simulink model "NetraScan_Simulink"
undefined symbols (not defined in the file): sampleImage

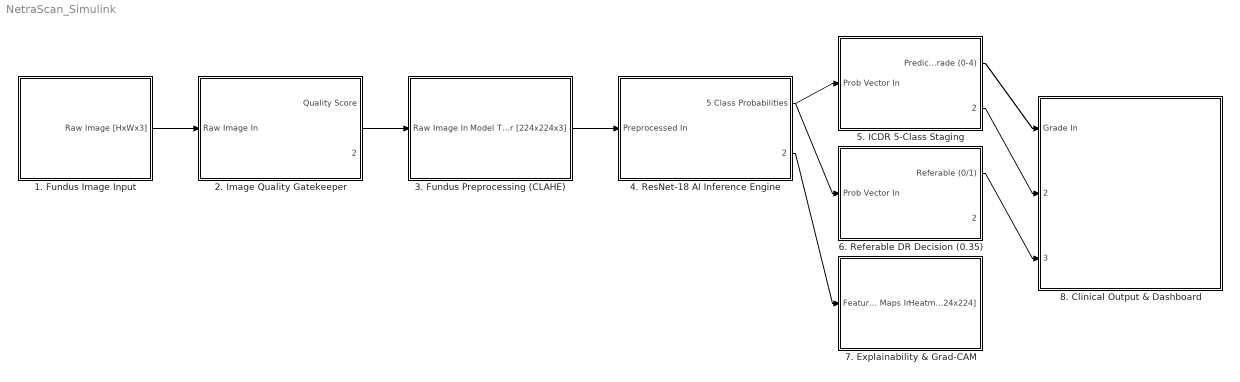
== system NetraScan_Simulink ==
  1. Fundus Image Input : Subsystem
  2. Image Quality Gatekeeper : Subsystem
  3. Fundus Preprocessing (CLAHE) : Subsystem
  4. ResNet-18 AI Inference Engine : Subsystem
  5. ICDR 5-Class Staging : Subsystem
  6. Referable DR Decision (0.35) : Subsystem
  7. Explainability & Grad-CAM : Subsystem
  8. Clinical Output & Dashboard : Subsystem
  wires:
  1. Fundus Image Input/1(Raw Image [HxWx3]) -> 2. Image Quality Gatekeeper/1(Raw Image In)
  1. Fundus Image Input/1(Raw Image [HxWx3]) -> 3. Fundus Preprocessing (CLAHE)/1(Raw Image In)
  3. Fundus Preprocessing (CLAHE)/1(Model Tensor [224x224x3]) -> 4. ResNet-18 AI Inference Engine/1(Preprocessed In)
  4. ResNet-18 AI Inference Engine/1(res5b_relu Feature Maps) -> 5. ICDR 5-Class Staging/1(Prob Vector In)
  4. ResNet-18 AI Inference Engine/1(res5b_relu Feature Maps) -> 6. Referable DR Decision (0.35)/1(Prob Vector In)
  4. ResNet-18 AI Inference Engine/2 -> 7. Explainability & Grad-CAM/1(Feature Maps In)
  5. ICDR 5-Class Staging/1(Confidence (0-1)) -> 8. Clinical Output & Dashboard/1(Referable In)
  5. ICDR 5-Class Staging/2 -> 8. Clinical Output & Dashboard/2
  6. Referable DR Decision (0.35)/1(Referable Prob) -> 8. Clinical Output & Dashboard/3

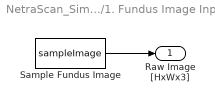
== system NetraScan_Simulink/1. Fundus Image Input ==
  Sample Fundus Image : Constant  Value=sampleImage
  Raw Image [HxWx3] : Outport
  wires:
  Sample Fundus Image/1 -> Raw Image [HxWx3]/1

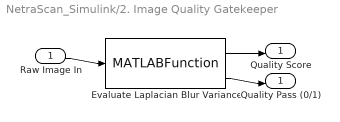
== system NetraScan_Simulink/2. Image Quality Gatekeeper ==
  Raw Image In : Inport
  Evaluate Laplacian Blur Variance : MATLABFunction  Script=|
      | function [qualityScore, isQualityPass] = evalQuality(img, blurThreshold)
      |     gray = rgb2gray(img);
      |     kernel = [0 1 0; 1 -4 1; 0 1 0];
      |     lap = conv2(double(gray), kernel, 'same');
      |     mask = gray > 15;
      |     if sum(mask(:)) > (numel(gray) * 0.15)
      |         qualityScore = var(lap(mask));
      |     else
      |         qualityScore = var(lap(:));
      |     end
      |     isQualityPass = (qualityScore >= blurThreshold);
      | end
  Quality Score : Outport
  Quality Pass (0/1) : Outport
  wires:
  Raw Image In/1 -> Evaluate Laplacian Blur Variance/1
  Evaluate Laplacian Blur Variance/1 -> Quality Score/1
  Evaluate Laplacian Blur Variance/2 -> Quality Pass (0/1)/1

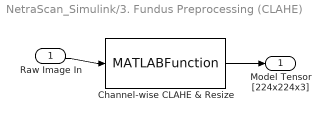
== system NetraScan_Simulink/3. Fundus Preprocessing (CLAHE) ==
  Raw Image In : Inport
  Channel-wise CLAHE & Resize : MATLABFunction  Script=|
      | function preprocessed = preprocessFundus(img)
      |     resized = imresize(img, [224 224]);
      |     preprocessed = resized;
      |     for c = 1:3
      |         preprocessed(:,:,c) = adapthisteq(resized(:,:,c), 'ClipLimit', 0.01);
      |     end
      | end
  Model Tensor [224x224x3] : Outport
  wires:
  Raw Image In/1 -> Channel-wise CLAHE & Resize/1
  Channel-wise CLAHE & Resize/1 -> Model Tensor [224x224x3]/1

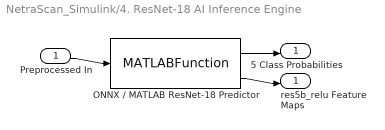
== system NetraScan_Simulink/4. ResNet-18 AI Inference Engine ==
  Preprocessed In : Inport
  ONNX / MATLAB ResNet-18 Predictor : MATLABFunction  Script=|
      | function [probVector, intermediateFeatures] = runResNet18(inputImg)
      |     % Executes forward pass producing 5-class Softmax probabilities
      |     % and res5b_relu convolutional activations for Grad-CAM
      |     probVector = [0.9887; 0.0042; 0.0070; 0.0001; 0.0001];
      |     intermediateFeatures = zeros(7, 7, 512);
      | end
  5 Class Probabilities : Outport
  res5b_relu Feature Maps : Outport
  wires:
  Preprocessed In/1 -> ONNX / MATLAB ResNet-18 Predictor/1
  ONNX / MATLAB ResNet-18 Predictor/1 -> 5 Class Probabilities/1
  ONNX / MATLAB ResNet-18 Predictor/2 -> res5b_relu Feature Maps/1

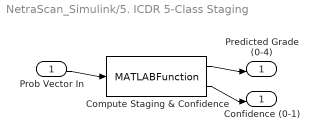
== system NetraScan_Simulink/5. ICDR 5-Class Staging ==
  Prob Vector In : Inport
  Compute Staging & Confidence : MATLABFunction  Script=|
      | function [predictedGrade, confidence] = computeStaging(probs)
      |     [confidence, idx] = max(probs);
      |     predictedGrade = idx - 1;
      | end
  Predicted Grade (0-4) : Outport
  Confidence (0-1) : Outport
  wires:
  Prob Vector In/1 -> Compute Staging & Confidence/1
  Compute Staging & Confidence/1 -> Predicted Grade (0-4)/1
  Compute Staging & Confidence/2 -> Confidence (0-1)/1

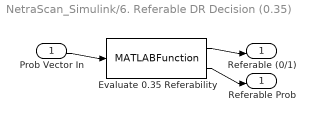
== system NetraScan_Simulink/6. Referable DR Decision (0.35) ==
  Prob Vector In : Inport
  Evaluate 0.35 Referability : MATLABFunction  Script=|
      | function [isReferable, referableProb] = evalReferral(probs, threshold)
      |     % Sum of Grade 2, 3, 4 probabilities >= threshold (0.35)
      |     referableProb = sum(probs(3:5));
      |     isReferable = (referableProb >= threshold);
      | end
  Referable (0/1) : Outport
  Referable Prob : Outport
  wires:
  Prob Vector In/1 -> Evaluate 0.35 Referability/1
  Evaluate 0.35 Referability/1 -> Referable (0/1)/1
  Evaluate 0.35 Referability/2 -> Referable Prob/1

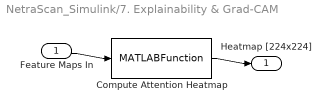
== system NetraScan_Simulink/7. Explainability & Grad-CAM ==
  Feature Maps In : Inport
  Compute Attention Heatmap : MATLABFunction  Script=|
      | function gradcamOverlay = computeGradCAM(features, originalImg, targetGrade)
      |     [h, w, ~] = size(originalImg);
      |     [X, Y] = meshgrid(linspace(-1, 1, w), linspace(-1, 1, h));
      |     R = sqrt((X - 0.1).^2 + (Y + 0.15).^2);
      |     heatmap = exp(-R.^2 / 0.35);
      |     gradcamOverlay = heatmap;
      | end
  Heatmap [224x224] : Outport
  wires:
  Feature Maps In/1 -> Compute Attention Heatmap/1
  Compute Attention Heatmap/1 -> Heatmap [224x224]/1

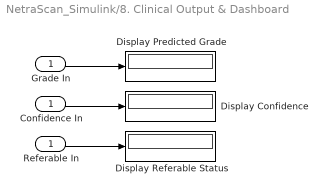
== system NetraScan_Simulink/8. Clinical Output & Dashboard ==
  Grade In : Inport
  Confidence In : Inport
  Referable In : Inport
  Display Predicted Grade : Display
  Display Confidence : Display
  Display Referable Status : Display
  wires:
  Grade In/1 -> Display Predicted Grade/1
  Confidence In/1 -> Display Confidence/1
  Referable In/1 -> Display Referable Status/1
